simulink model "masasprezynasimulink"  (R2018b)
settings: Solver=FixedStepAuto  StartTime=0.0  StopTime=tk  FixedStep=dt  RelTol=1e-3
values from neighbouring files (symbols this model uses):
  c1 = 0.2    [Wywolawczy.m]    (also in Wywolawczy2.m; Wywolawczy3.m; Wywolawczy4.m; Wywolawczy5.m)
  c2 = 1    [Wywolawczy.m]    (also in Wywolawczy2.m; Wywolawczy3.m; Wywolawczy4.m; Wywolawczy5.m)
  dt = 1e-2    (= 0.01)    [plikwykon.m]
  k1 = 2    [Wywolawczy.m]    (also in Wywolawczy2.m; Wywolawczy3.m; Wywolawczy4.m; Wywolawczy5.m)
  k2 = 2    [Wywolawczy.m]    (also in Wywolawczy2.m; Wywolawczy3.m; Wywolawczy4.m; Wywolawczy5.m)
  m1 = 3    [Wywolawczy.m]    (also in Wywolawczy2.m; Wywolawczy3.m; Wywolawczy4.m; Wywolawczy5.m)
  m2 = 0.5    [Wywolawczy.m]    (also in Wywolawczy2.m; Wywolawczy3.m; Wywolawczy4.m; Wywolawczy5.m)
undefined symbols (not defined in the file or in its folder): DiscIntNeverNeededParam
settings Model: Creator=user  LastModifiedBy=juan

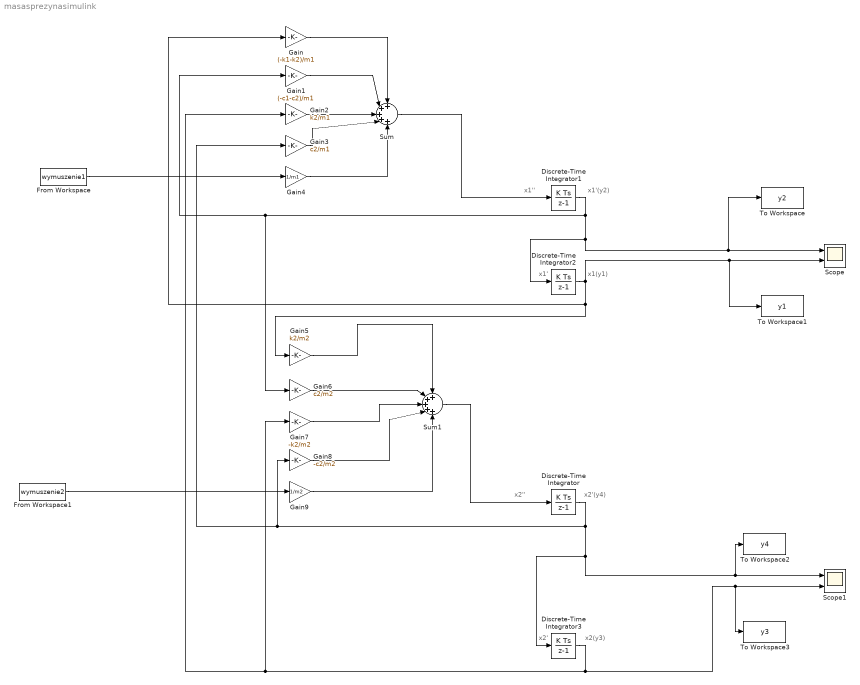
== system masasprezynasimulink ==
  note: x2''
  note: x1''
  note: x1'
  note: x1'(y2)
  note: x1(y1)
  note: x2'(y4)
  note: x2'
  note: x2(y3)
  Discrete-Time Integrator{,1..3} (4 alike) : DiscreteIntegrator  SampleTime=dt  ICPrevOutput=DiscIntNeverNeededParam  ICPrevScaledInput=DiscIntNeverNeededParam
  From Workspace : FromWorkspace  VariableName=wymuszenie1  SampleTime=dt
  From Workspace1 : FromWorkspace  VariableName=wymuszenie2  SampleTime=dt
  Gain : Gain  Gain=(-k1-k2)/m1
  Gain1 : Gain  Gain=(-c1-c2)/m1
  Gain2 : Gain  Gain=k2/m1
  Gain3 : Gain  Gain=c2/m1
  Gain4 : Gain  Gain=1/m1
  Gain5 : Gain  Gain=k2/m2
  Gain6 : Gain  Gain=c2/m2
  Gain7 : Gain  Gain=-k2/m2
  Gain8 : Gain  Gain=-c2/m2
  Gain9 : Gain  Gain=1/m2
  Scope : Scope  NumInputPorts=2
  Scope1 : Scope  NumInputPorts=2
  Sum : Sum  Inputs=+++++
  Sum1 : Sum  Inputs=+++++
  To Workspace : ToWorkspace  VariableName=y2  SampleTime=dt
      settings: Save2DSignal=2-D array (concatenate along first dimension)
  To Workspace1 : ToWorkspace  VariableName=y1  SampleTime=dt
      settings: Save2DSignal=2-D array (concatenate along first dimension)
  To Workspace2 : ToWorkspace  VariableName=y4  SampleTime=dt
      settings: Save2DSignal=2-D array (concatenate along first dimension)
  To Workspace3 : ToWorkspace  VariableName=y3  SampleTime=dt
      settings: Save2DSignal=2-D array (concatenate along first dimension)
  wires:
  Discrete-Time Integrator1/1 -> Gain6/1, Gain1/1, To Workspace/1, Scope/1, Discrete-Time Integrator2/1
  Discrete-Time Integrator/1 -> To Workspace2/1, Scope1/1, Discrete-Time Integrator3/1, Gain3/1, Gain8/1
  Sum/1 -> Discrete-Time Integrator1/1
  Gain/1 -> Sum/1
  Discrete-Time Integrator2/1 -> Gain5/1, Gain/1, To Workspace1/1, Scope/2
  Gain1/1 -> Sum/2
  Gain2/1 -> Sum/3
  Discrete-Time Integrator3/1 -> Gain7/1, Gain2/1, To Workspace3/1, Scope1/2
  Gain3/1 -> Sum/4
  Gain4/1 -> Sum/5
  From Workspace/1 -> Gain4/1
  Sum1/1 -> Discrete-Time Integrator/1
  Gain5/1 -> Sum1/1
  Gain6/1 -> Sum1/2
  Gain7/1 -> Sum1/3
  Gain8/1 -> Sum1/4
  Gain9/1 -> Sum1/5
  From Workspace1/1 -> Gain9/1
